simulink model "DisplacementObserver_basicModel"  (R2017a)
settings: Solver=VariableStepAuto  StartTime=0.0  StopTime=5  MaxStep=0.001  RelTol=1e-6
values from neighbouring files (symbols this model uses):
  a1 = mlg/J    (= 22.3011494253)    [InitParams.m]
  b1 = -k/J    (= -0.377011494253)    [InitParams.m]
  curLoopKI = R/desiredTCur    (= 202.666666667)    [InitParams.m]
  curLoopKP = L/desiredTCur    (= 1)    [InitParams.m]
  dTheta0 = 1    [InitParams.m]
  dThetaRW0 = -1    [InitParams.m]
  J = Jp + mp*lp*lp + mr*lr*lr    (= 0.097875)    [InitParams.m]
  Jr = 8e-04    (= 0.0008)    [InitParams.m]
  k = 0.0369    [InitParams.m]
  Klqr = lqr(Alin,Blin,Qlqr,Rlqr)    [InitParams.m]
  L = 0.003    [InitParams.m]
  Lobs = [546;1100;-508]    [InitParams.m]
  mechParams = [J, Jr, Cp, Cr, mlg]    [InitParams.m]
  mlg = (mp*lp + mr*lr)*g    (= 2.182725)    [InitParams.m]
  R = 0.608    [InitParams.m]
  theta0 = -0.1    [InitParams.m]
  thetaDisplacement = 0.1    [InitParams.m]
  thetaRW0 = 0    [InitParams.m]
  Umax = 24    [InitParams.m]
undefined symbols (not defined in the file): ap, ar, kp, kr, xp0, xr0
settings Model: Creator=aranovskiy_sta  LastModifiedBy=Stas

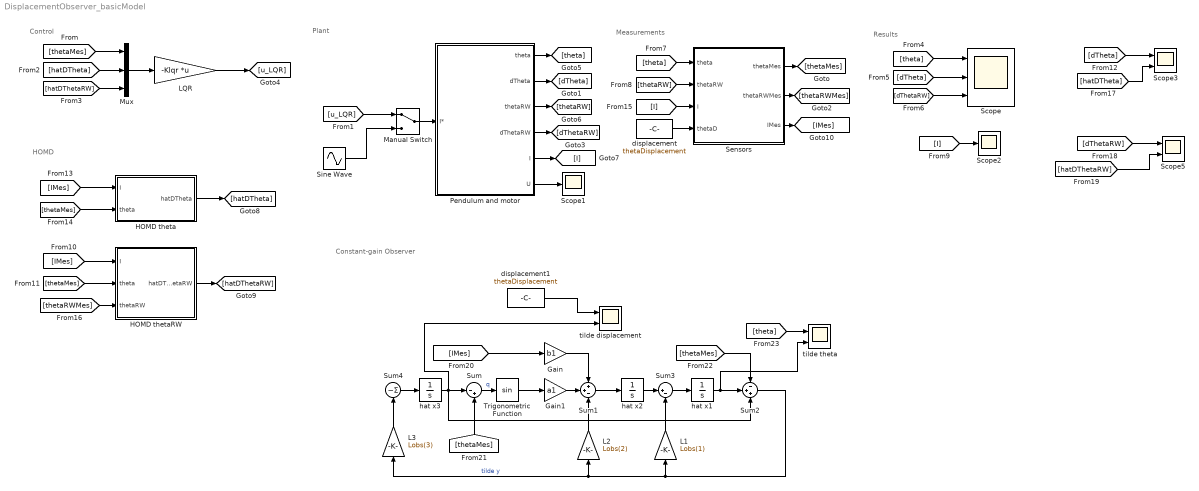
== system DisplacementObserver_basicModel ==
  note: Constant-gain Observer
  note: Plant
  note: Measurements
  note: Control
  note: Results
  note: HOMD
  Gain : Gain  Gain=b1
  Gain1 : Gain  Gain=a1
  HOMD theta : Subsystem  mask{a=ap, k=kp, x0=xp0, kTorque=k, mlg=mlg, J=J}
      mask prompts: a "alpha"; k "gains K"; x0 "Initial value"; kTorque "torque constant"; J "Inertia"
      mask DialogControl DescTextVar Prompt: HOMD for theta
      mask DialogControl Container3 Prompt: Mech params
  HOMD thetaRW : Subsystem  mask{a=ar, k=kr, x0=xr0, kTorque=k, mlg=mlg, J=J, Jr=Jr}
      mask prompts: a "alpha"; k "gains K"; x0 "Initial value"; kTorque "torque constant"; J "Inertia"
      mask DialogControl DescTextVar Prompt: HOMD for thetaRW
      mask DialogControl Container3 Prompt: Mech params
  L1 : Gain  Gain=Lobs(1)
  L2 : Gain  Gain=Lobs(2)
  L3 : Gain  Gain=Lobs(3)
  LQR : Gain  Gain=-Klqr  Multiplication=Matrix(K*u)
  Manual Switch : ManualSwitch
  Mux : Mux  Inputs=3
  Pendulum and motor : Subsystem
  Scope : Scope  NumInputPorts=3
  Scope1 : Scope
  Scope2 : Scope
  Scope3 : Scope  NumInputPorts=2
  Scope5 : Scope  NumInputPorts=2
  Sensors : Subsystem
  Sine Wave : Sin  Frequency=3  SampleTime=0
  Sum : Sum  Inputs=|-+
  Sum1 : Sum  Inputs=++-
  Sum2 : Sum  Inputs=-++
  Sum3 : Sum  Inputs=|+-
  Sum4 : Sum  Inputs=||-
  Trigonometric Function : Trigonometry
  displacement : Constant  Value=thetaDisplacement
  displacement1 : Constant  Value=thetaDisplacement
  hat x1 : Integrator
  hat x2 : Integrator
  hat x3 : Integrator  LimitOutput=on  UpperSaturationLimit=0.5  LowerSaturationLimit=-0.5
  tilde displacement : Scope  NumInputPorts=2
  tilde theta : Scope  NumInputPorts=2
  wires:
  [thetaMes] -> Mux/1
  [hatDTheta] -> Mux/2
  [hatDThetaRW] -> Mux/3
  Mux/1 -> LQR/1
  LQR/1 -> [u_LQR]
  [theta] -> Scope/1
  [dTheta] -> Scope/2
  [dThetaRW] -> Scope/3
  Pendulum and motor/1(theta) -> [theta]
  Sensors/1(thetaMes) -> [thetaMes]
  Pendulum and motor/2(dTheta) -> [dTheta]
  Sensors/2(thetaRWMes) -> [thetaRWMes]
  Pendulum and motor/4(dThetaRW) -> [dThetaRW]
  Pendulum and motor/3(thetaRW) -> [thetaRW]
  [theta] -> Sensors/1(theta)
  [thetaRW] -> Sensors/2(thetaRW)
  [u_LQR] -> Manual Switch/1
  Manual Switch/1 -> Pendulum and motor/1(I*)
  Sine Wave/1 -> Manual Switch/2
  Pendulum and motor/5(I) -> [I]
  Pendulum and motor/6(U) -> Scope1/1
  [I] -> Scope2/1
  [dTheta] -> Scope3/1
  [thetaRWMes] -> HOMD thetaRW/3(thetaRW)
  HOMD theta/1(hatDTheta) -> [hatDTheta]
  [hatDTheta] -> Scope3/2
  [dThetaRW] -> Scope5/1
  [hatDThetaRW] -> Scope5/2
  HOMD thetaRW/1(hatDThetaRW) -> [hatDThetaRW]
  [I] -> Sensors/3(I)
  Sensors/3(IMes) -> [IMes]
  [IMes] -> HOMD theta/1(I)
  [thetaMes] -> HOMD theta/2(theta)
  [IMes] -> HOMD thetaRW/1(I)
  [thetaMes] -> HOMD thetaRW/2(theta)
  displacement/1 -> Sensors/4(thetaD)
  [IMes] -> Gain/1
  Sum/1 -> Trigonometric Function/1  "q"
  Trigonometric Function/1 -> Gain1/1
  Gain/1 -> Sum1/1
  [thetaMes] -> Sum2/1
  Sum2/1 -> L1/1, L3/1, L2/1  "tilde y"
  hat x1/1 -> tilde theta/2, Sum2/2
  Sum1/1 -> hat x2/1
  hat x2/1 -> Sum3/1
  Sum3/1 -> hat x1/1
  L1/1 -> Sum3/2
  L2/1 -> Sum1/3
  [thetaMes] -> Sum/2
  hat x3/1 -> Sum2/3, tilde displacement/2, Sum/1
  Sum4/1 -> hat x3/1
  L3/1 -> Sum4/1
  displacement1/1 -> tilde displacement/1
  [theta] -> tilde theta/1
  Gain1/1 -> Sum1/2

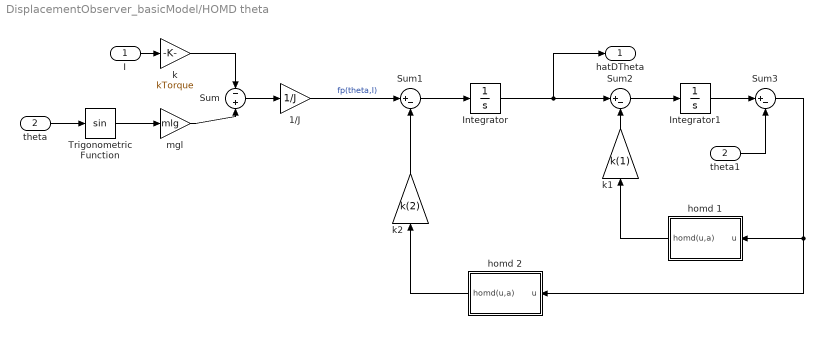
== system DisplacementObserver_basicModel/HOMD theta ==
  I : Inport
  theta : Inport  Port=2
  1/J : Gain  Gain=1/J
  Integrator : Integrator  InitialCondition=x0(2)
  Integrator1 : Integrator  InitialCondition=x0(1)
  Sum : Sum  Inputs=-+
  Sum1 : Sum  Inputs=|+-
  Sum2 : Sum  Inputs=|+-
  Sum3 : Sum  Inputs=|+-
  Trigonometric Function : Trigonometry
  homd 1 : Subsystem  mask{alpha=a}
      mask DialogControl q Prompt: homd(u,a) = sign(u)*abs(u)^a
  homd 2 : Subsystem  mask{alpha=2*a-1}
      mask DialogControl q Prompt: homd(u,a) = sign(u)*abs(u)^a
  k : Gain  Gain=kTorque
  k1 : Gain  Gain=k(1)
  k2 : Gain  Gain=k(2)
  mgl : Gain  Gain=mlg
  theta1 : InportShadow  Port=2
  hatDTheta : Outport
  wires:
  1/J/1 -> Sum1/1  "fp(theta,I)"
  Integrator/1 -> hatDTheta/1, Sum2/1
  k/1 -> Sum/1
  Trigonometric Function/1 -> mgl/1
  Sum/1 -> 1/J/1
  Sum2/1 -> Integrator1/1
  Integrator1/1 -> Sum3/1
  Sum1/1 -> Integrator/1
  k2/1 -> Sum1/2
  k1/1 -> Sum2/2
  mgl/1 -> Sum/2
  theta1/1 -> Sum3/2
  theta/1 -> Trigonometric Function/1
  Sum3/1 -> homd 2/1(u), homd 1/1(u)
  I/1 -> k/1
  homd 2/1(homd(u,a)) -> k2/1
  homd 1/1(homd(u,a)) -> k1/1

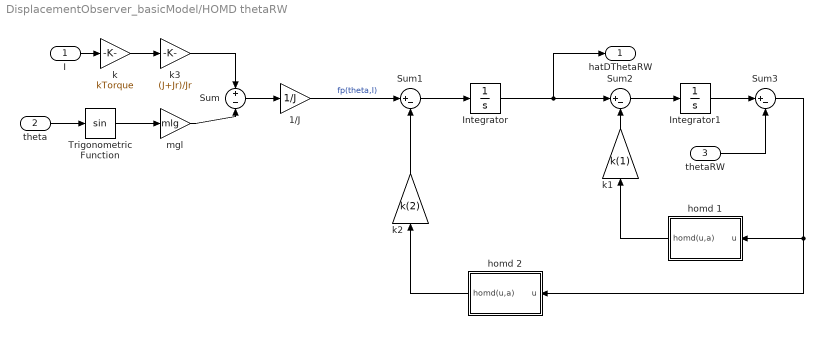
== system DisplacementObserver_basicModel/HOMD thetaRW ==
  I : Inport
  theta : Inport  Port=2
  thetaRW : Inport  Port=3
  1/J : Gain  Gain=1/J
  Integrator : Integrator  InitialCondition=x0(2)
  Integrator1 : Integrator  InitialCondition=x0(1)
  Sum : Sum  Inputs=+-
  Sum1 : Sum  Inputs=|+-
  Sum2 : Sum  Inputs=|+-
  Sum3 : Sum  Inputs=|+-
  Trigonometric Function : Trigonometry
  homd 1 : Subsystem  mask{alpha=a}
      mask DialogControl q Prompt: homd(u,a) = sign(u)*abs(u)^a
  homd 2 : Subsystem  mask{alpha=2*a-1}
      mask DialogControl q Prompt: homd(u,a) = sign(u)*abs(u)^a
  k : Gain  Gain=kTorque
  k1 : Gain  Gain=k(1)
  k2 : Gain  Gain=k(2)
  k3 : Gain  Gain=(J+Jr)/Jr
  mgl : Gain  Gain=mlg
  hatDThetaRW : Outport
  wires:
  homd 1/1(homd(u,a)) -> k1/1
  homd 2/1(homd(u,a)) -> k2/1
  I/1 -> k/1
  Sum3/1 -> homd 1/1(u), homd 2/1(u)
  theta/1 -> Trigonometric Function/1
  mgl/1 -> Sum/2
  k1/1 -> Sum2/2
  k2/1 -> Sum1/2
  Sum1/1 -> Integrator/1
  Integrator1/1 -> Sum3/1
  Sum2/1 -> Integrator1/1
  Sum/1 -> 1/J/1
  Trigonometric Function/1 -> mgl/1
  Integrator/1 -> Sum2/1, hatDThetaRW/1
  1/J/1 -> Sum1/1  "fp(theta,I)"
  thetaRW/1 -> Sum3/2
  k/1 -> k3/1
  k3/1 -> Sum/1

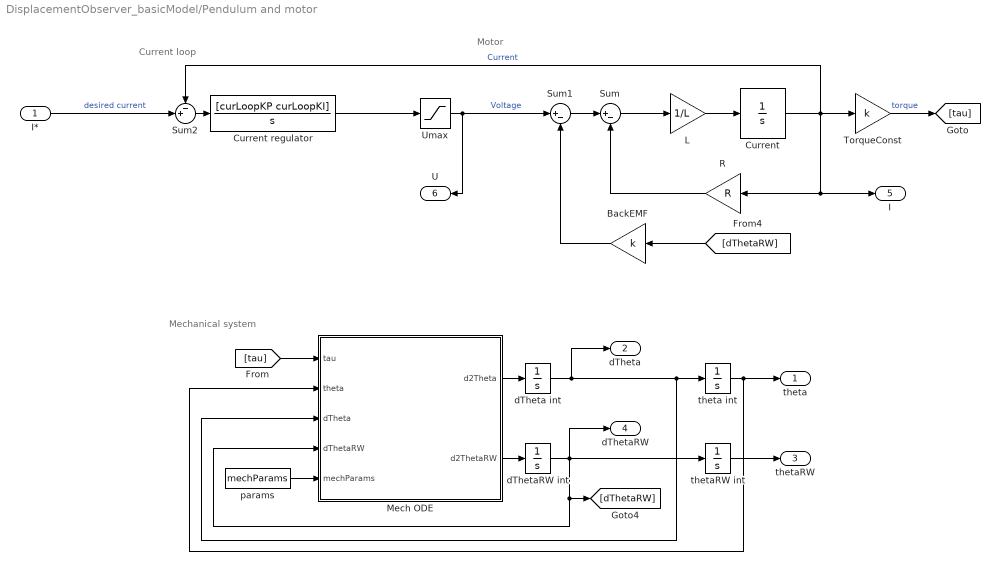
== system DisplacementObserver_basicModel/Pendulum and motor ==
  note: Mechanical system
  note: Current loop
  note: Motor
  I* : Inport
  BackEMF : Gain  Gain=k
  Current : Integrator
  Current regulator : TransferFcn  Numerator=[curLoopKP curLoopKI]  Denominator=[1 0]
  L : Gain  Gain=1/L
  Mech ODE : MATLAB Function  TreatAsAtomicUnit=on
  R : Gain  Gain=R
  Sum : Sum  Inputs=|+-
  Sum1 : Sum  Inputs=|+-
  Sum2 : Sum  Inputs=-+|
  TorqueConst : Gain  Gain=k
  Umax : Saturate  UpperLimit=Umax  LowerLimit=-Umax
  dTheta int : Integrator  InitialCondition=dTheta0
  dThetaRW int : Integrator  InitialCondition=dThetaRW0
  params : Constant  Value=mechParams
  theta int : Integrator  InitialCondition=theta0
  thetaRW int : Integrator  InitialCondition=thetaRW0
  theta : Outport
  dTheta : Outport  Port=2
  thetaRW : Outport  Port=3
  dThetaRW : Outport  Port=4
  I : Outport  Port=5
  U : Outport  Port=6
  wires:
  Sum/1 -> L/1
  L/1 -> Current/1
  Sum1/1 -> Sum/1
  BackEMF/1 -> Sum1/2
  Sum2/1 -> Current regulator/1
  R/1 -> Sum/2
  Umax/1 -> U/1, Sum1/1  "Voltage"
  Current regulator/1 -> Umax/1
  Current/1 -> I/1, R/1, Sum2/1, TorqueConst/1  "Current"
  params/1 -> Mech ODE/5(mechParams)
  Mech ODE/2(d2ThetaRW) -> dThetaRW int/1
  TorqueConst/1 -> [tau]  "torque"
  Mech ODE/1(d2Theta) -> dTheta int/1
  dTheta int/1 -> dTheta/1, Mech ODE/3(dTheta), theta int/1
  [dThetaRW] -> BackEMF/1
  [tau] -> Mech ODE/1(tau)
  dThetaRW int/1 -> dThetaRW/1, Mech ODE/4(dThetaRW), [dThetaRW], thetaRW int/1
  theta int/1 -> theta/1, Mech ODE/2(theta)
  thetaRW int/1 -> thetaRW/1
  I*/1 -> Sum2/2  "desired current"

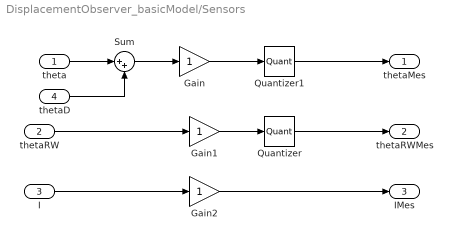
== system DisplacementObserver_basicModel/Sensors ==
  theta : Inport
  thetaRW : Inport  Port=2
  I : Inport  Port=3
  thetaD : Inport  Port=4
  Gain : Gain
  Gain1 : Gain
  Gain2 : Gain
  Quantizer : Quantizer  QuantizationInterval=2*pi/48
  Quantizer1 : Quantizer  QuantizationInterval=2*pi/10000
  Sum : Sum  Inputs=|++
  thetaMes : Outport
  thetaRWMes : Outport  Port=2
  IMes : Outport  Port=3
  wires:
  thetaRW/1 -> Gain1/1
  Gain1/1 -> Quantizer/1
  Gain/1 -> Quantizer1/1
  I/1 -> Gain2/1
  Gain2/1 -> IMes/1
  Quantizer/1 -> thetaRWMes/1
  Quantizer1/1 -> thetaMes/1
  Sum/1 -> Gain/1
  thetaD/1 -> Sum/2
  theta/1 -> Sum/1

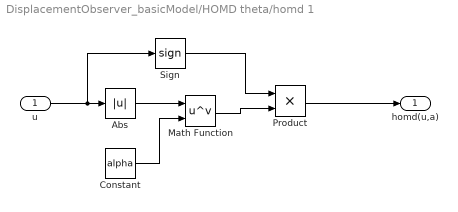
== system DisplacementObserver_basicModel/HOMD theta/homd 1 ==
  u : Inport
  Abs : Abs
  Constant : Constant  Value=alpha
  Math Function : Math  Operator=pow  SaturateOnIntegerOverflow=on
  Product : Product
  Sign : Signum
  homd(u,a) : Outport
  wires:
  Sign/1 -> Product/1
  Product/1 -> homd(u,a)/1
  Constant/1 -> Math Function/2
  Math Function/1 -> Product/2
  u/1 -> Sign/1, Abs/1
  Abs/1 -> Math Function/1

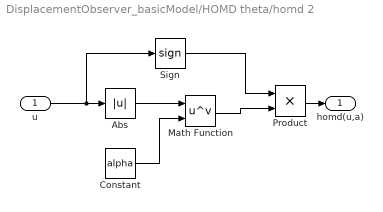
== system DisplacementObserver_basicModel/HOMD theta/homd 2 ==
  u : Inport
  Abs : Abs
  Constant : Constant  Value=alpha
  Math Function : Math  Operator=pow  SaturateOnIntegerOverflow=on
  Product : Product
  Sign : Signum
  homd(u,a) : Outport
  wires:
  Abs/1 -> Math Function/1
  u/1 -> Abs/1, Sign/1
  Math Function/1 -> Product/2
  Constant/1 -> Math Function/2
  Product/1 -> homd(u,a)/1
  Sign/1 -> Product/1

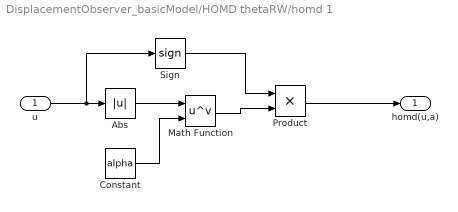
== system DisplacementObserver_basicModel/HOMD thetaRW/homd 1 ==
  u : Inport
  Abs : Abs
  Constant : Constant  Value=alpha
  Math Function : Math  Operator=pow  SaturateOnIntegerOverflow=on
  Product : Product
  Sign : Signum
  homd(u,a) : Outport
  wires:
  Abs/1 -> Math Function/1
  u/1 -> Abs/1, Sign/1
  Math Function/1 -> Product/2
  Constant/1 -> Math Function/2
  Product/1 -> homd(u,a)/1
  Sign/1 -> Product/1

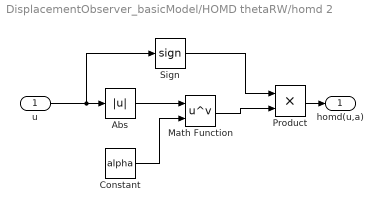
== system DisplacementObserver_basicModel/HOMD thetaRW/homd 2 ==
  u : Inport
  Abs : Abs
  Constant : Constant  Value=alpha
  Math Function : Math  Operator=pow  SaturateOnIntegerOverflow=on
  Product : Product
  Sign : Signum
  homd(u,a) : Outport
  wires:
  Sign/1 -> Product/1
  Product/1 -> homd(u,a)/1
  Constant/1 -> Math Function/2
  Math Function/1 -> Product/2
  u/1 -> Sign/1, Abs/1
  Abs/1 -> Math Function/1

== matlab function DisplacementObserver_basicModel/Pendulum and motor/Mech ODE ==
  data: tau input; theta input; d2Theta output; dTheta input; dThetaRW input; mechParams input; d2ThetaRW output
function [d2Theta, d2ThetaRW] = RWPendODE(tau, theta, dTheta, dThetaRW, mechParams)
%RWODE Compute the derivatives

% The parameters are: J, Jr, Cp, Cr, R, k, Umax, mlg

J = mechParams(1);
Jr = mechParams(2);
Cp = mechParams(3);
Cr = mechParams(4);
mlg = mechParams(5);

% The model    
M = [Jr Jr; Jr J+Jr];
G = [0; -mlg*sin(theta)];
T = [-Cr*dThetaRW+tau; -Cp*dTheta];

d2q=M\(-G+T);

d2Theta=d2q(2);
d2ThetaRW=d2q(1);
end
